simulink model "GMCLIB_SvmStd_BAM_FLT"  (Simulink 8.3)
settings: Solver=ode45  StartTime=0.0  StopTime=10.0  RelTol=1e-3
settings Model: Creator=RE004C  LastModifiedBy=B17364
settings OptimizationCC: ExpressionDepthLimit=2147483647
settings DebuggingCC: FcnCallInpInsideContextMsg=UseLocalSettings  StrictBusMsg=Warning
settings HardwareCC: ProdLargestAtomicInteger=Long  ProdLargestAtomicFloat=Double  ProdIntDivRoundTo=Zero  ProdEndianess=BigEndian  ProdHWDeviceType=Freescale->32-bit PowerPC

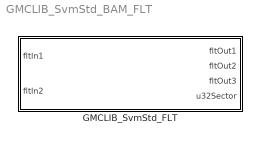
== system GMCLIB_SvmStd_BAM_FLT ==
  GMCLIB_SvmStd_FLT : Subsystem  mask(GMCLIB_SvmStd_FLT){}
      mask help: Bit accurate model of Standard Space Vector Modulation.
      mask init:
      | pos = get_param(gcb, 'Position');width = pos(3) - pos(1); height = pos(4) - pos(2);tX=width/2;tY=height*0.9;
      mask Display: color('black');port_label('input',1,'fltIn1');port_label('input',2,'fltIn2');port_label('output',1,'fltOut1');port_label('output',2,'fltOut2');port_label('output',3,'fltOut3');port_label('output',4,'u32Sector');color('black');disp('GMCLIB_SvmStd_FLT');color('blue');text(tX,tY, 'BAM', 'horizontalAlignment', 'center');

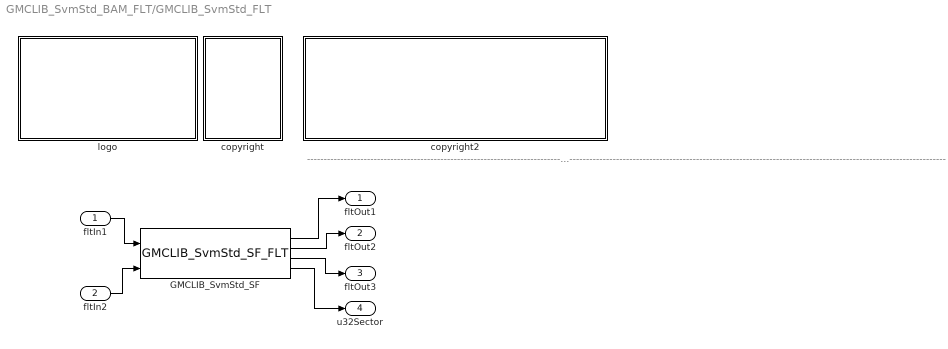
== system GMCLIB_SvmStd_BAM_FLT/GMCLIB_SvmStd_FLT ==
  note: ---------------------------------------------------------------------------------------------------------------------------------------------------------------------------------------------------
  fltIn1 : Inport
  fltIn2 : Inport  Port=2
  GMCLIB_SvmStd_SF : S-Function  FunctionName=GMCLIB_SvmStd_SF_FLT  EnableBusSupport=off
  copyright : Subsystem
      mask Display:
      | text(10,90,'FILE:');text(10,75,'DESRIPTION:')
      | text(10,60,'COPYRIGHT:')
      | text(10,45,'VERSION:')
      | text(10,30,'DATE:')
  copyright2 : Subsystem
      mask Display:
      | text(10,90,'GMCLIB_SvmStd_BAM_FLT.mdl');text(10,75,'Standard Space Vector Modulation.');text(10,60,'Freescale')
      | text(10,45,'0.1');text(10,30,'26-Sep-2011');
  logo : Subsystem
      mask Display: image(imread('logo.jpg'))
  fltOut1 : Outport
  fltOut2 : Outport  Port=2
  fltOut3 : Outport  Port=3
  u32Sector : Outport  Port=4
  wires:
  fltIn1/1 -> GMCLIB_SvmStd_SF/1
  fltIn2/1 -> GMCLIB_SvmStd_SF/2
  GMCLIB_SvmStd_SF/1 -> fltOut1/1
  GMCLIB_SvmStd_SF/2 -> fltOut2/1
  GMCLIB_SvmStd_SF/3 -> fltOut3/1
  GMCLIB_SvmStd_SF/4 -> u32Sector/1

== system GMCLIB_SvmStd_BAM_FLT/GMCLIB_SvmStd_FLT/copyright ==

== system GMCLIB_SvmStd_BAM_FLT/GMCLIB_SvmStd_FLT/copyright2 ==

== system GMCLIB_SvmStd_BAM_FLT/GMCLIB_SvmStd_FLT/logo ==
